simulink model "cic2"  (Simulink 8.1)
settings: Solver=ode3  StartTime=0.0  StopTime=1  FixedStep=1/fs  RelTol=1e-3
values from neighbouring files (symbols this model uses):
  fs = sq_wave_freq*osr    (= 10000000)    [param2.m]
libraries: dspsigops x2
settings Model: Creator=hp  LastModifiedBy=amr

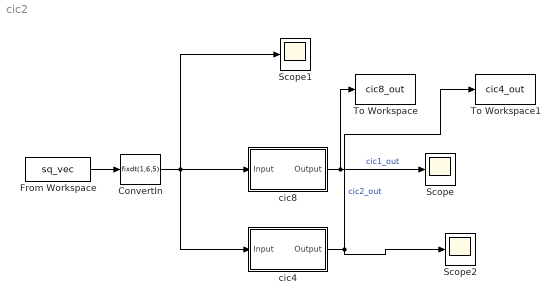
== system cic2 ==
  ConvertIn : DataTypeConversion  OutDataTypeStr=fixdt(1,6,5)  RndMeth=Nearest  SaturateOnIntegerOverflow=on
  From Workspace : FromWorkspace  VariableName=sq_vec  SampleTime=1/fs  Interpolate=off  OutputAfterFinalValue=Holding final value
  Scope : Scope
  Scope1 : Scope
  Scope2 : Scope
      settings: SaveName=ScopeData2
  To Workspace : ToWorkspace  VariableName=cic8_out  SampleTime=-1
  To Workspace1 : ToWorkspace  VariableName=cic4_out  SampleTime=-1
  cic4 : Subsystem  Tag=FilterWizardSubSystem
      settings: ErrorFcn=dspFilterRealizedInBasicElemsAlgLoopErrFcnCallback
  cic8 : Subsystem  Tag=FilterWizardSubSystem
      settings: ErrorFcn=dspFilterRealizedInBasicElemsAlgLoopErrFcnCallback
  wires:
  From Workspace/1 -> ConvertIn/1
  cic8/1(Output) -> To Workspace/1, Scope/1  "cic1_out"
  cic4/1(Output) -> Scope2/1, To Workspace1/1  "cic2_out"
  ConvertIn/1 -> cic4/1(Input), cic8/1(Input), Scope1/1

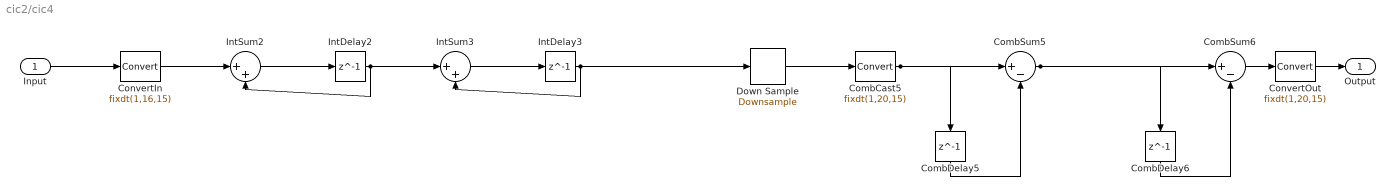
== system cic2/cic4 ==
  Input : Inport
  CombCast5 : DataTypeConversion  OutDataTypeStr=fixdt(1,20,15)
  CombDelay5 : Delay  DelayLength=1  InitialCondition=0
  CombDelay6 : Delay  DelayLength=1  InitialCondition=0
  CombSum5 : Sum  Inputs=|+-  AccumDataTypeStr=fixdt(1,20,15)  OutDataTypeStr=fixdt(1,20,15)
  CombSum6 : Sum  Inputs=|+-  AccumDataTypeStr=fixdt(1,20,15)  OutDataTypeStr=fixdt(1,20,15)
  ConvertIn : DataTypeConversion  OutDataTypeStr=fixdt(1,16,15)  RndMeth=Nearest  SaturateOnIntegerOverflow=on
  ConvertOut : DataTypeConversion  OutDataTypeStr=fixdt(1,20,15)
  Down Sample : dspsigops/Downsample  N=4  phase=0  RateOptions=Allow multirate processing  smode=Allow multirate  fmode=Maintain input frame size  ic=0
  IntDelay2 : Delay  DelayLength=1  InitialCondition=0
  IntDelay3 : Delay  DelayLength=1  InitialCondition=0
  IntSum2 : Sum  Inputs=|++  AccumDataTypeStr=fixdt(1,20,15)  OutDataTypeStr=fixdt(1,20,15)
  IntSum3 : Sum  Inputs=|++  AccumDataTypeStr=fixdt(1,20,15)  OutDataTypeStr=fixdt(1,20,15)
  Output : Outport
  wires:
  Input/1 -> ConvertIn/1
  ConvertIn/1 -> IntSum2/1
  IntSum2/1 -> IntDelay2/1
  IntDelay2/1 -> IntSum2/2, IntSum3/1
  IntSum3/1 -> IntDelay3/1
  IntDelay3/1 -> IntSum3/2, Down Sample/1
  Down Sample/1 -> CombCast5/1
  CombSum5/1 -> CombSum6/1, CombDelay6/1
  CombDelay5/1 -> CombSum5/2
  CombCast5/1 -> CombSum5/1, CombDelay5/1
  CombSum6/1 -> ConvertOut/1
  CombDelay6/1 -> CombSum6/2
  ConvertOut/1 -> Output/1

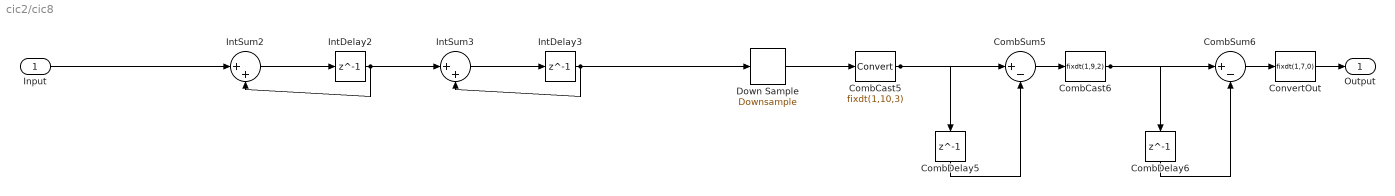
== system cic2/cic8 ==
  Input : Inport
  CombCast5 : DataTypeConversion  OutDataTypeStr=fixdt(1,10,3)
  CombCast6 : DataTypeConversion  OutDataTypeStr=fixdt(1,9,2)
  CombDelay5 : Delay  DelayLength=1  InitialCondition=0
  CombDelay6 : Delay  DelayLength=1  InitialCondition=0
  CombSum5 : Sum  Inputs=|+-  AccumDataTypeStr=fixdt(1,10,3)  OutDataTypeStr=fixdt(1,10,3)
  CombSum6 : Sum  Inputs=|+-  AccumDataTypeStr=fixdt(1,9,2)  OutDataTypeStr=fixdt(1,9,2)  SaturateOnIntegerOverflow=on
  ConvertOut : DataTypeConversion  OutDataTypeStr=fixdt(1,7,0)
  Down Sample : dspsigops/Downsample  N=8  phase=0  RateOptions=Allow multirate processing  smode=Allow multirate  fmode=Maintain input frame size  ic=0
  IntDelay2 : Delay  DelayLength=1  InitialCondition=0
  IntDelay3 : Delay  DelayLength=1  InitialCondition=0
  IntSum2 : Sum  Inputs=|++  AccumDataTypeStr=fixdt(1,12,5)  OutDataTypeStr=fixdt(1,12,5)
  IntSum3 : Sum  Inputs=|++  AccumDataTypeStr=fixdt(1,10,3)  OutDataTypeStr=fixdt(1,10,3)
  Output : Outport
  wires:
  Input/1 -> IntSum2/1
  IntSum2/1 -> IntDelay2/1
  IntDelay2/1 -> IntSum2/2, IntSum3/1
  IntSum3/1 -> IntDelay3/1
  IntDelay3/1 -> IntSum3/2, Down Sample/1
  Down Sample/1 -> CombCast5/1
  CombSum5/1 -> CombCast6/1
  CombDelay5/1 -> CombSum5/2
  CombCast5/1 -> CombSum5/1, CombDelay5/1
  CombSum6/1 -> ConvertOut/1
  CombDelay6/1 -> CombSum6/2
  CombCast6/1 -> CombSum6/1, CombDelay6/1
  ConvertOut/1 -> Output/1
